simulink model "pmsm_ideal"  (Simulink 9.3)
settings: Solver=ode23tb  StartTime=0.0  StopTime=0.12  MaxStep=0.00001  RelTol=1e-4  EnableMultiTasking=on
settings Model: Creator=jagan  LastModifiedBy=Administrator
settings SolverCC: ZeroCrossAlgorithm=Non-adaptive
settings DataIOCC: LimitDataPoints=on  SignalLoggingName=sigsOut
settings OptimizationCC: ExpressionDepthLimit=2147483647  InitFltsAndDblsToZero=on
settings DebuggingCC: SaveWithParameterizedLinksMsg=none  SignalResolutionControl=TryResolveAllWithWarning  MultiTaskDSMMsg=warning  MultiTaskCondExecSysMsg=none  StateNameClashWarn=warning
settings HardwareCC: TargetUnknown=on
settings SFSimCC: SimUseLocalCustomCode=on
settings RTWCC: RTWUseLocalCustomCode=on
settings ConfigComp: CovExternalEMLEnable=on

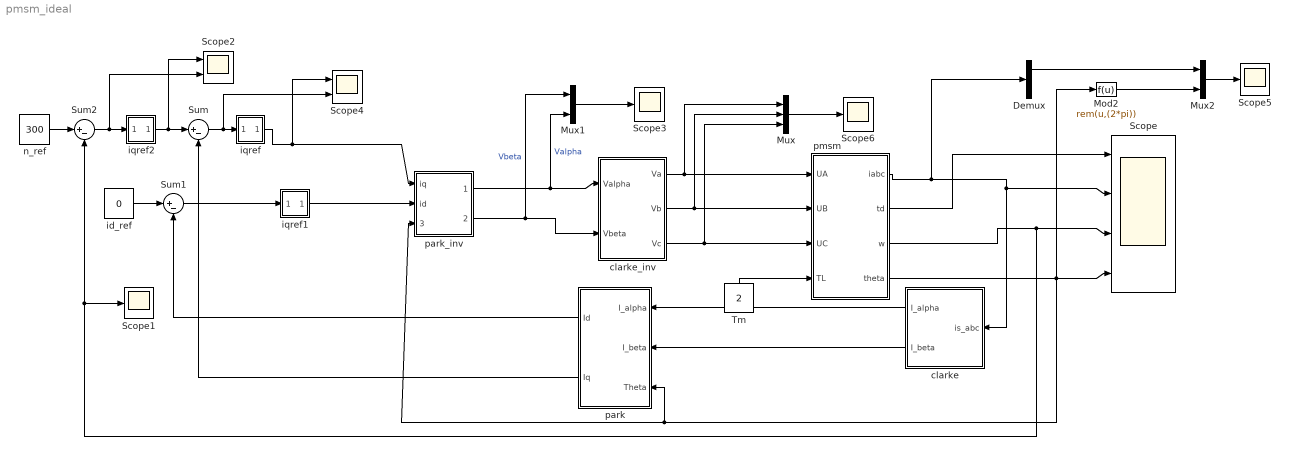
== system pmsm_ideal ==
  Demux : Demux  Outputs=3
  Mod2 : Fcn  Expr=rem(u,(2*pi))
  Mux : Mux  Inputs=3
  Mux1 : Mux  Inputs=2
  Mux2 : Mux  Inputs=2
  Scope : Scope  NumInputPorts=4
  Scope{1,3,5..6} (4 alike) : Scope
  Scope2 : Scope  NumInputPorts=2
  Scope4 : Scope  NumInputPorts=2
  Sum : Sum  Inputs=|+-  SaturateOnIntegerOverflow=on
  Sum1 : Sum  Inputs=|+-  SaturateOnIntegerOverflow=on
  Sum2 : Sum  Inputs=|+-  SaturateOnIntegerOverflow=on
  Tm : Constant  Value=2
  clarke : Subsystem
  clarke_inv : Subsystem
  id_ref : Constant  Value=0
  iqref : Subsystem  mask(PI Controller){I=5, P=10, sat=[-500, 500]}
      mask prompts: I "Integral"; P "Proportional:"; sat "Minimum and maximum outputs:"
      mask init:
      | min=sat(1);max=sat(2);
      mask Display: disp('PI')
  iqref1 : Subsystem  mask(PI Controller){I=5, P=10, sat=[-500, 500]}
      mask prompts: I "Integral"; P "Proportional:"; sat "Minimum and maximum outputs:"
      mask init:
      | min=sat(1);max=sat(2);
      mask Display: disp('PI')
  iqref2 : Subsystem  mask(PI Controller){I=5, P=10, sat=[-30, 30]}
      mask prompts: I "Integral"; P "Proportional:"; sat "Minimum and maximum outputs:"
      mask init:
      | min=sat(1);max=sat(2);
      mask Display: disp('PI')
  n_ref : Constant  Value=300
  park : Subsystem
  park_inv : Subsystem
  pmsm : Subsystem  mask(hao){CL=0.175, Pm=4, Ld=0.0085, Lq=0.0085, rs=2.875*0.1, J=0.0008}
      mask help: pmsm
      mask Help: no
  wires:
  Sum/1 -> iqref/1(In_1), Scope4/2
  iqref2/1(Out_1) -> Sum/1, Scope2/1
  park/2(Iq) -> Sum/2
  park/1(Id) -> Sum1/2
  id_ref/1 -> Sum1/1
  Sum2/1 -> iqref2/1(In_1), Scope2/2
  n_ref/1 -> Sum2/1
  Tm/1 -> pmsm/4(TL)
  clarke/1(I_alpha) -> park/1(I_alpha)
  clarke/2(I_beta) -> park/2(I_beta)
  Sum1/1 -> iqref1/1(In_1)
  pmsm/1(iabc) -> Demux/1, Scope/2, clarke/1(is_abc)
  pmsm/3(w) -> Sum2/2, Scope1/1, Scope/3
  Mux/1 -> Scope6/1
  iqref/1(Out_1) -> Scope4/1, park_inv/1(iq)
  pmsm/2(td) -> Scope/1
  park_inv/2(I_beta) -> clarke_inv/2(Vbeta), Mux1/1  "Vbeta"
  park_inv/1(I_apha) -> clarke_inv/1(Valpha), Mux1/2  "Valpha"
  pmsm/4(theta) -> Mod2/1, park/3(Theta), park_inv/3(Theta), Scope/4
  clarke_inv/1(Va) -> pmsm/1(UA), Mux/1
  clarke_inv/2(Vb) -> pmsm/2(UB), Mux/2
  clarke_inv/3(Vc) -> pmsm/3(UC), Mux/3
  Mux1/1 -> Scope3/1
  iqref1/1(Out_1) -> park_inv/2(id)
  Demux/1 -> Mux2/1
  Mux2/1 -> Scope5/1
  Mod2/1 -> Mux2/2

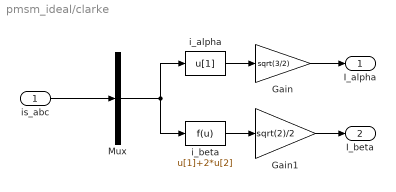
== system pmsm_ideal/clarke ==
  is_abc : Inport
  Gain : Gain  Gain=sqrt(3/2)  SaturateOnIntegerOverflow=on  OutDataTypeStr=Inherit: Same as input  ParamDataTypeStr=Inherit: Same as input
  Gain1 : Gain  Gain=sqrt(2)/2  SaturateOnIntegerOverflow=on  OutDataTypeStr=Inherit: Same as input  ParamDataTypeStr=Inherit: Same as input
  Mux : Mux  Inputs=[3]
  i_alpha : Fcn  Expr=u[1]
  i_beta : Fcn  Expr=u[1]+2*u[2]
  I_alpha : Outport  InitialOutput=0
  I_beta : Outport  Port=2  InitialOutput=0
  wires:
  Mux/1 -> i_beta/1, i_alpha/1
  is_abc/1 -> Mux/1
  i_beta/1 -> Gain1/1
  i_alpha/1 -> Gain/1
  Gain/1 -> I_alpha/1
  Gain1/1 -> I_beta/1

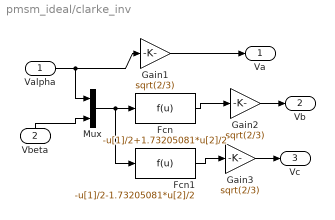
== system pmsm_ideal/clarke_inv ==
  Valpha : Inport
  Vbeta : Inport  Port=2
  Fcn : Fcn  Expr=-u[1]/2+1.73205081*u[2]/2
  Fcn1 : Fcn  Expr=-u[1]/2-1.73205081*u[2]/2
  Gain1 : Gain  Gain=sqrt(2/3)  SaturateOnIntegerOverflow=on  OutDataTypeStr=Inherit: Same as input  ParamDataTypeStr=Inherit: Same as input
  Gain2 : Gain  Gain=sqrt(2/3)  SaturateOnIntegerOverflow=on  OutDataTypeStr=Inherit: Same as input  ParamDataTypeStr=Inherit: Same as input
  Gain3 : Gain  Gain=sqrt(2/3)  SaturateOnIntegerOverflow=on  OutDataTypeStr=Inherit: Same as input  ParamDataTypeStr=Inherit: Same as input
  Mux : Mux  Inputs=2
  Va : Outport
  Vb : Outport  Port=2
  Vc : Outport  Port=3
  wires:
  Mux/1 -> Fcn/1, Fcn1/1
  Fcn/1 -> Gain2/1
  Fcn1/1 -> Gain3/1
  Valpha/1 -> Gain1/1, Mux/1
  Vbeta/1 -> Mux/2
  Gain1/1 -> Va/1
  Gain2/1 -> Vb/1
  Gain3/1 -> Vc/1

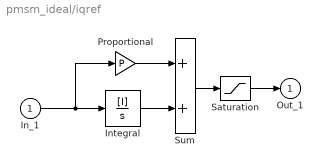
== system pmsm_ideal/iqref ==
  In_1 : Inport
  Integral : TransferFcn  Numerator=[I]  Denominator=[1 0]
  Proportional : Gain  Gain=P  SaturateOnIntegerOverflow=on  OutDataTypeStr=Inherit: Same as input  ParamDataTypeStr=Inherit: Same as input
  Saturation : Saturate  UpperLimit=max  LowerLimit=min
  Sum : Sum  SaturateOnIntegerOverflow=on  InputSameDT=on  OutDataTypeStr=Inherit: Same as first input
  Out_1 : Outport  InitialOutput=0
  wires:
  Integral/1 -> Sum/2
  In_1/1 -> Integral/1, Proportional/1
  Proportional/1 -> Sum/1
  Sum/1 -> Saturation/1
  Saturation/1 -> Out_1/1

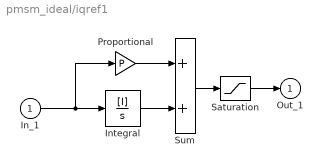
== system pmsm_ideal/iqref1 ==
  In_1 : Inport
  Integral : TransferFcn  Numerator=[I]  Denominator=[1 0]
  Proportional : Gain  Gain=P  SaturateOnIntegerOverflow=on  OutDataTypeStr=Inherit: Same as input  ParamDataTypeStr=Inherit: Same as input
  Saturation : Saturate  UpperLimit=max  LowerLimit=min
  Sum : Sum  SaturateOnIntegerOverflow=on  InputSameDT=on  OutDataTypeStr=Inherit: Same as first input
  Out_1 : Outport  InitialOutput=0
  wires:
  Saturation/1 -> Out_1/1
  Sum/1 -> Saturation/1
  Proportional/1 -> Sum/1
  In_1/1 -> Proportional/1, Integral/1
  Integral/1 -> Sum/2

== system pmsm_ideal/iqref2 ==
  In_1 : Inport
  Integral : TransferFcn  Numerator=[I]  Denominator=[1 0]
  Proportional : Gain  Gain=P  SaturateOnIntegerOverflow=on  OutDataTypeStr=Inherit: Same as input  ParamDataTypeStr=Inherit: Same as input
  Saturation : Saturate  UpperLimit=max  LowerLimit=min
  Sum : Sum  SaturateOnIntegerOverflow=on  InputSameDT=on  OutDataTypeStr=Inherit: Same as first input
  Out_1 : Outport  InitialOutput=0
  wires:
  Saturation/1 -> Out_1/1
  Sum/1 -> Saturation/1
  Proportional/1 -> Sum/1
  In_1/1 -> Proportional/1, Integral/1
  Integral/1 -> Sum/2

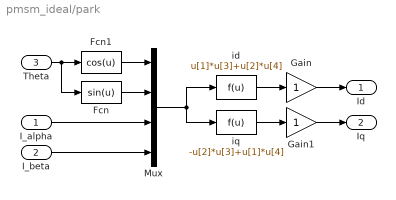
== system pmsm_ideal/park ==
  I_alpha : Inport
  I_beta : Inport  Port=2
  Theta : Inport  Port=3
  Fcn : Fcn  Expr=sin(u)
  Fcn1 : Fcn  Expr=cos(u)
  Gain : Gain  SaturateOnIntegerOverflow=on  OutDataTypeStr=Inherit: Same as input  ParamDataTypeStr=Inherit: Same as input
  Gain1 : Gain  SaturateOnIntegerOverflow=on  OutDataTypeStr=Inherit: Same as input  ParamDataTypeStr=Inherit: Same as input
  Mux : Mux  Inputs=[1 1 1 1]
  id : Fcn  Expr=u[1]*u[3]+u[2]*u[4]
  iq : Fcn  Expr=-u[2]*u[3]+u[1]*u[4]
  Id : Outport  InitialOutput=0
  Iq : Outport  Port=2  InitialOutput=0
  wires:
  Fcn/1 -> Mux/2
  Fcn1/1 -> Mux/1
  Theta/1 -> Fcn1/1, Fcn/1
  Mux/1 -> iq/1, id/1
  I_alpha/1 -> Mux/3
  iq/1 -> Gain1/1
  id/1 -> Gain/1
  Gain/1 -> Id/1
  Gain1/1 -> Iq/1
  I_beta/1 -> Mux/4

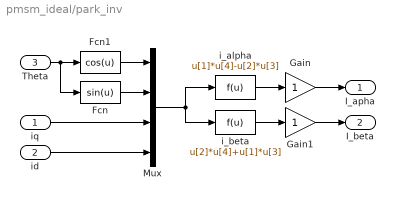
== system pmsm_ideal/park_inv ==
  iq : Inport
  id : Inport  Port=2
  Theta : Inport  Port=3
  Fcn : Fcn  Expr=sin(u)
  Fcn1 : Fcn  Expr=cos(u)
  Gain : Gain  SaturateOnIntegerOverflow=on  OutDataTypeStr=Inherit: Same as input  ParamDataTypeStr=Inherit: Same as input
  Gain1 : Gain  SaturateOnIntegerOverflow=on  OutDataTypeStr=Inherit: Same as input  ParamDataTypeStr=Inherit: Same as input
  Mux : Mux  Inputs=[1 1 1 1]
  i_alpha : Fcn  Expr=u[1]*u[4]-u[2]*u[3]
  i_beta : Fcn  Expr=u[2]*u[4]+u[1]*u[3]
  I_apha : Outport  InitialOutput=0
  I_beta : Outport  Port=2  InitialOutput=0
  wires:
  Fcn/1 -> Mux/2
  Fcn1/1 -> Mux/1
  Theta/1 -> Fcn1/1, Fcn/1
  Mux/1 -> i_beta/1, i_alpha/1
  iq/1 -> Mux/3
  i_beta/1 -> Gain1/1
  i_alpha/1 -> Gain/1
  Gain/1 -> I_apha/1
  Gain1/1 -> I_beta/1
  id/1 -> Mux/4

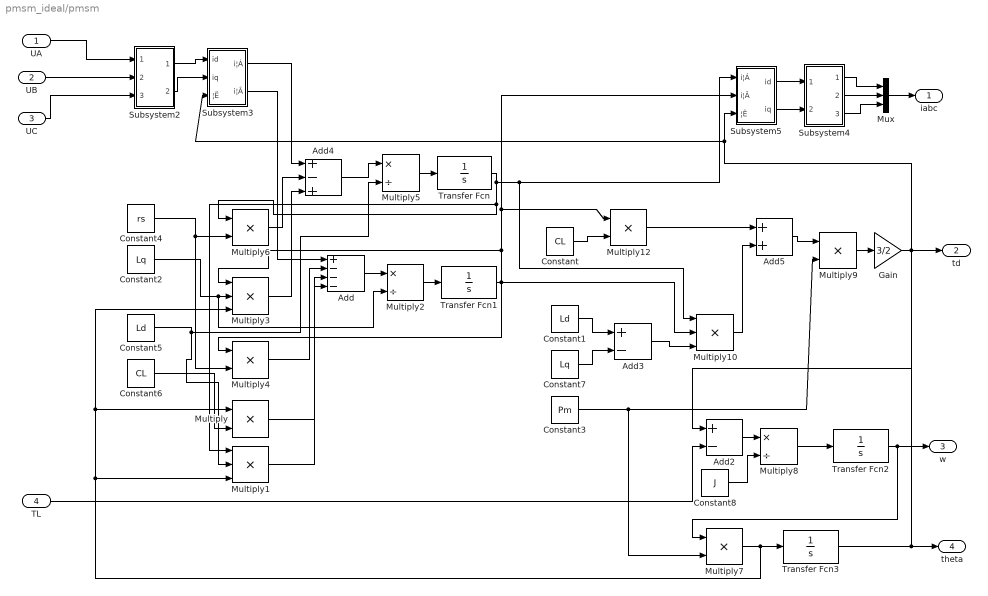
== system pmsm_ideal/pmsm ==
  UA : Inport
  UB : Inport  Port=2
  UC : Inport  Port=3
  TL : Inport  Port=4
  Add : Sum  Inputs=+---  SaturateOnIntegerOverflow=on  OutDataTypeStr=Inherit: Same as first input
  Add2 : Sum  Inputs=+-  SaturateOnIntegerOverflow=on  InputSameDT=on  OutDataTypeStr=Inherit: Same as first input
  Add3 : Sum  Inputs=+-  SaturateOnIntegerOverflow=on  InputSameDT=on  OutDataTypeStr=Inherit: Same as first input
  Add4 : Sum  Inputs=+-+  SaturateOnIntegerOverflow=on  InputSameDT=on  OutDataTypeStr=Inherit: Same as first input
  Add5 : Sum  SaturateOnIntegerOverflow=on  InputSameDT=on  OutDataTypeStr=Inherit: Same as first input
  Constant : Constant  Value=CL
  Constant1 : Constant  Value=Ld
  Constant2 : Constant  Value=Lq
  Constant3 : Constant  Value=Pm
  Constant4 : Constant  Value=rs
  Constant5 : Constant  Value=Ld
  Constant6 : Constant  Value=CL
  Constant7 : Constant  Value=Lq
  Constant8 : Constant  Value=J
  Gain : Gain  Gain=3/2  SaturateOnIntegerOverflow=on  OutDataTypeStr=Inherit: Same as input  ParamDataTypeStr=Inherit: Same as input
  Multiply{,4,6..7,9,12} (6 alike) : Product  Inputs=**  SaturateOnIntegerOverflow=on  OutDataTypeStr=Inherit: Same as first input
  Multiply1 : Product  Inputs=***  SaturateOnIntegerOverflow=on  OutDataTypeStr=Inherit: Same as first input
  Multiply10 : Product  Inputs=***  SaturateOnIntegerOverflow=on  OutDataTypeStr=Inherit: Same as first input
  Multiply2 : Product  Inputs=*/  SaturateOnIntegerOverflow=on  OutDataTypeStr=Inherit: Same as first input
  Multiply3 : Product  Inputs=***  SaturateOnIntegerOverflow=on  OutDataTypeStr=Inherit: Same as first input
  Multiply5 : Product  Inputs=*/  SaturateOnIntegerOverflow=on  OutDataTypeStr=Inherit: Same as first input
  Multiply8 : Product  Inputs=*/  SaturateOnIntegerOverflow=on  OutDataTypeStr=Inherit: Same as first input
  Mux : Mux  Inputs=3
  Subsystem2 : Subsystem  mask(hao){}
      mask help: 3/2
      mask Help: no
      mask Display: disp('3/2')
  Subsystem3 : Subsystem  mask(2/2){}
      mask help: qdtoMT
      mask Help: none
  Subsystem4 : Subsystem  mask(hao){}
      mask help: 2/3
      mask Help: npi
      mask Display: disp('2/3')
  Subsystem5 : Subsystem  mask(2/2){}
      mask help: mt-todq
      mask Help: no
  Transfer Fcn : TransferFcn  Denominator=[1 0]  AbsoluteTolerance=1e-3
  Transfer Fcn1 : TransferFcn  Denominator=[1 0]
  Transfer Fcn2 : TransferFcn  Denominator=[1 0]
  Transfer Fcn3 : TransferFcn  Denominator=[1 0]
  iabc : Outport
  td : Outport  Port=2
  w : Outport  Port=3
  theta : Outport  Port=4
  wires:
  Multiply2/1 -> Transfer Fcn1/1
  Multiply5/1 -> Transfer Fcn/1
  TL/1 -> Add2/2
  Constant8/1 -> Multiply8/2
  Add2/1 -> Multiply8/1
  Subsystem5/2(iq) -> Subsystem4/2(In3)
  Subsystem5/1(id) -> Subsystem4/1(In1)
  Constant3/1 -> Multiply7/2, Multiply9/2
  Multiply10/1 -> Add5/2
  Multiply12/1 -> Add5/1
  Constant7/1 -> Add3/2
  Constant1/1 -> Add3/1
  Multiply1/1 -> Add/4
  Multiply/1 -> Add/3
  Multiply4/1 -> Add/2
  Add/1 -> Multiply2/1
  Subsystem3/2(i¦Â) -> Add/1
  Add4/1 -> Multiply5/1
  Multiply3/1 -> Add4/3
  Multiply6/1 -> Add4/2
  Subsystem3/1(i¦Á) -> Add4/1
  Subsystem2/2(Out2) -> Subsystem3/2(iq)
  Subsystem2/1(Out1) -> Subsystem3/1(id)
  Transfer Fcn/1 -> Multiply6/1, Multiply1/1, Multiply10/1, Subsystem5/1(i¦Á)
  Constant4/1 -> Multiply6/2, Multiply4/2
  Transfer Fcn1/1 -> Multiply3/1, Multiply12/1, Subsystem5/2(i¦Â), Multiply4/1, Multiply10/2
  Constant2/1 -> Multiply3/2, Multiply2/2
  Constant5/1 -> Multiply1/2, Multiply5/2
  Constant6/1 -> Multiply/2
  Multiply7/1 -> Transfer Fcn3/1, Multiply3/3, Multiply/1, Multiply1/3
  Constant/1 -> Multiply12/2
  Add3/1 -> Multiply10/3
  Transfer Fcn2/1 -> Multiply7/1, w/1
  Add5/1 -> Multiply9/1
  Multiply9/1 -> Gain/1
  Subsystem4/3(Out3) -> Mux/3
  Mux/1 -> iabc/1
  Multiply8/1 -> Transfer Fcn2/1
  UC/1 -> Subsystem2/3(In3)
  Transfer Fcn3/1 -> Subsystem5/3(¦Ë), Subsystem3/3(¦Ë), theta/1
  Gain/1 -> td/1, Add2/1
  Subsystem4/1(Out1) -> Mux/1
  Subsystem4/2(Out2) -> Mux/2
  UA/1 -> Subsystem2/1(In1)
  UB/1 -> Subsystem2/2(In2)

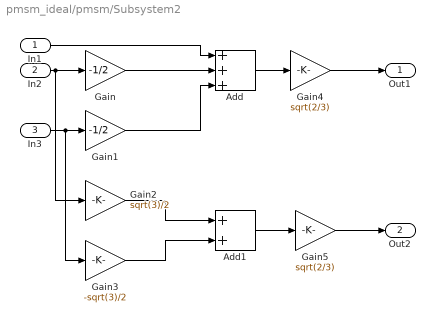
== system pmsm_ideal/pmsm/Subsystem2 ==
  In1 : Inport
  In2 : Inport  Port=2
  In3 : Inport  Port=3
  Add : Sum  Inputs=+++  SaturateOnIntegerOverflow=on  InputSameDT=on  OutDataTypeStr=Inherit: Same as first input
  Add1 : Sum  SaturateOnIntegerOverflow=on  InputSameDT=on  OutDataTypeStr=Inherit: Same as first input
  Gain : Gain  Gain=-1/2  SaturateOnIntegerOverflow=on  OutDataTypeStr=Inherit: Same as input  ParamDataTypeStr=Inherit: Same as input
  Gain1 : Gain  Gain=-1/2  SaturateOnIntegerOverflow=on  OutDataTypeStr=Inherit: Same as input  ParamDataTypeStr=Inherit: Same as input
  Gain2 : Gain  Gain=sqrt(3)/2  SaturateOnIntegerOverflow=on  OutDataTypeStr=Inherit: Same as input  ParamDataTypeStr=Inherit: Same as input
  Gain3 : Gain  Gain=-sqrt(3)/2  SaturateOnIntegerOverflow=on  OutDataTypeStr=Inherit: Same as input  ParamDataTypeStr=Inherit: Same as input
  Gain4 : Gain  Gain=sqrt(2/3)  SaturateOnIntegerOverflow=on  OutDataTypeStr=Inherit: Same as input  ParamDataTypeStr=Inherit: Same as input
  Gain5 : Gain  Gain=sqrt(2/3)  SaturateOnIntegerOverflow=on  OutDataTypeStr=Inherit: Same as input  ParamDataTypeStr=Inherit: Same as input
  Out1 : Outport
  Out2 : Outport  Port=2
  wires:
  Gain5/1 -> Out2/1
  Gain4/1 -> Out1/1
  Add1/1 -> Gain5/1
  In3/1 -> Gain3/1, Gain1/1
  In2/1 -> Gain2/1, Gain/1
  Add/1 -> Gain4/1
  In1/1 -> Add/1
  Gain3/1 -> Add1/2
  Gain2/1 -> Add1/1
  Gain1/1 -> Add/3
  Gain/1 -> Add/2

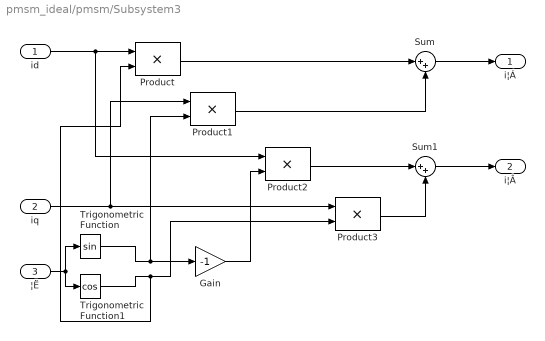
== system pmsm_ideal/pmsm/Subsystem3 ==
  id : Inport
  iq : Inport  Port=2
  ¦Ë : Inport  Port=3
  Gain : Gain  Gain=-1  SaturateOnIntegerOverflow=on  OutDataTypeStr=Inherit: Same as input  ParamDataTypeStr=Inherit: Same as input
  Product{,1..3} (4 alike) : Product  SaturateOnIntegerOverflow=on  OutDataTypeStr=Inherit: Same as first input
  Sum : Sum  Inputs=|++  SaturateOnIntegerOverflow=on  InputSameDT=on  OutDataTypeStr=Inherit: Same as first input
  Sum1 : Sum  Inputs=|++  SaturateOnIntegerOverflow=on  InputSameDT=on  OutDataTypeStr=Inherit: Same as first input
  Trigonometric Function : Trigonometry
  Trigonometric Function1 : Trigonometry  Operator=cos
  i¦Á : Outport
  i¦Â : Outport  Port=2
  wires:
  Product3/1 -> Sum1/2
  Product1/1 -> Sum/2
  Gain/1 -> Product2/2
  Trigonometric Function/1 -> Product1/2, Gain/1
  Trigonometric Function1/1 -> Product/2, Product3/2
  ¦Ë/1 -> Trigonometric Function1/1, Trigonometric Function/1
  iq/1 -> Product3/1, Product1/1
  Sum1/1 -> i¦Â/1
  Product2/1 -> Sum1/1
  Sum/1 -> i¦Á/1
  Product/1 -> Sum/1
  id/1 -> Product/1, Product2/1

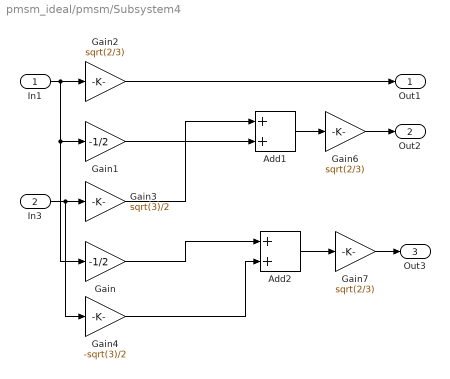
== system pmsm_ideal/pmsm/Subsystem4 ==
  In1 : Inport
  In3 : Inport  Port=2
  Add1 : Sum  SaturateOnIntegerOverflow=on  InputSameDT=on  OutDataTypeStr=Inherit: Same as first input
  Add2 : Sum  SaturateOnIntegerOverflow=on  InputSameDT=on  OutDataTypeStr=Inherit: Same as first input
  Gain : Gain  Gain=-1/2  SaturateOnIntegerOverflow=on  OutDataTypeStr=Inherit: Same as input  ParamDataTypeStr=Inherit: Same as input
  Gain1 : Gain  Gain=-1/2  SaturateOnIntegerOverflow=on  OutDataTypeStr=Inherit: Same as input  ParamDataTypeStr=Inherit: Same as input
  Gain2 : Gain  Gain=sqrt(2/3)  SaturateOnIntegerOverflow=on  OutDataTypeStr=Inherit: Same as input  ParamDataTypeStr=Inherit: Same as input
  Gain3 : Gain  Gain=sqrt(3)/2  SaturateOnIntegerOverflow=on  OutDataTypeStr=Inherit: Same as input  ParamDataTypeStr=Inherit: Same as input
  Gain4 : Gain  Gain=-sqrt(3)/2  SaturateOnIntegerOverflow=on  OutDataTypeStr=Inherit: Same as input  ParamDataTypeStr=Inherit: Same as input
  Gain6 : Gain  Gain=sqrt(2/3)  SaturateOnIntegerOverflow=on  OutDataTypeStr=Inherit: Same as input  ParamDataTypeStr=Inherit: Same as input
  Gain7 : Gain  Gain=sqrt(2/3)  SaturateOnIntegerOverflow=on  OutDataTypeStr=Inherit: Same as input  ParamDataTypeStr=Inherit: Same as input
  Out1 : Outport
  Out2 : Outport  Port=2
  Out3 : Outport  Port=3
  wires:
  Gain7/1 -> Out3/1
  In3/1 -> Gain4/1, Gain3/1
  Gain6/1 -> Out2/1
  Gain2/1 -> Out1/1
  In1/1 -> Gain/1, Gain1/1, Gain2/1
  Add2/1 -> Gain7/1
  Add1/1 -> Gain6/1
  Gain4/1 -> Add2/2
  Gain/1 -> Add2/1
  Gain3/1 -> Add1/2
  Gain1/1 -> Add1/1

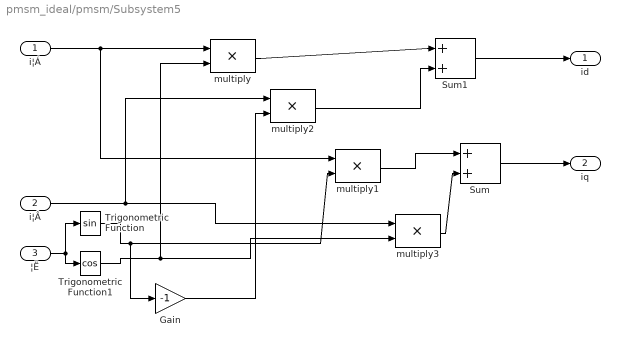
== system pmsm_ideal/pmsm/Subsystem5 ==
  i¦Á : Inport
  i¦Â : Inport  Port=2
  ¦Ë : Inport  Port=3
  Gain : Gain  Gain=-1  SaturateOnIntegerOverflow=on  OutDataTypeStr=Inherit: Same as input  ParamDataTypeStr=Inherit: Same as input
  Sum : Sum  Inputs=|++  SaturateOnIntegerOverflow=on  OutDataTypeStr=Inherit: Same as first input
  Sum1 : Sum  Inputs=|++  SaturateOnIntegerOverflow=on  OutDataTypeStr=Inherit: Same as first input
  Trigonometric Function : Trigonometry
  Trigonometric Function1 : Trigonometry  Operator=cos
  multiply{,1..3} (4 alike) : Product  SaturateOnIntegerOverflow=on  OutDataTypeStr=Inherit: Same as first input
  id : Outport
  iq : Outport  Port=2
  wires:
  ¦Ë/1 -> Trigonometric Function/1, Trigonometric Function1/1
  multiply/1 -> Sum1/1
  Sum1/1 -> id/1
  Sum/1 -> iq/1
  i¦Á/1 -> multiply1/1, multiply/1
  multiply1/1 -> Sum/1
  i¦Â/1 -> multiply2/1, multiply3/1
  multiply2/1 -> Sum1/2
  multiply3/1 -> Sum/2
  Trigonometric Function1/1 -> multiply3/2, multiply/2
  Trigonometric Function/1 -> multiply1/2, Gain/1
  Gain/1 -> multiply2/2
